simulink model "c_simulink"  (R2020a)
settings: Solver=VariableStepAuto  StartTime=0.0  StopTime=10  RelTol=1e-3
settings Model: Creator=jiw19031  LastModifiedBy=Amyang
settings OptimizationCC: BlockReduction=off  SimCompilerOptimization=on
settings ModelReferenceCC: UpdateModelReferenceTargets=Force
settings SFSimCC: SimCustomHeaderCode="#include \"tcpclient.h\""  SimUserSources=c/tcpclient.c  SimUserIncludeDirs=c/  SimUserLibraries=c/libws2_32.a  SimBuildMode=sf_nonincremental_build

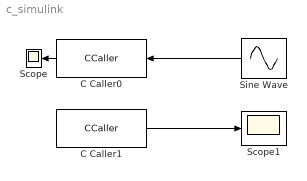
== system c_simulink ==
  C Caller0 : CCaller  FunctionName=TCPSend  PortSpecificationStruct="%)30     .    N ,   8    (     @         %    \"     (    !     0         %  0 \"0    $    _    07)G3F%M90  4&]R=$YA;64 4V-O<&4     26YD97@     5'EP90      4VEZ90      27-';&]B86P   X    P    !@    @    $          4    (     0    ,    !         !   P!O=70 #@   #     &    \"     0         !0    @    !     P    $         $  # &]U=  .    .     8    (    !          %    \"     $    &     0         0    !@   $]U='!U=   #@   #@    &    \"     8         !0    @    !     0    $         \"0    @               X    X    !@    @    $          4    (     0    8    !         !     &    9&]U8FQE   .    ,     8    (    !          %    \"     $    !     0         0  $ ,0    X    P    !@    @    ) @        4    (     0    $    !          (  0      #@   #     &    \"     0         !0    @    !     P    $         $  # &EN,  .    ,     8    (    !          %    \"     $    #     0         0  , :6XP  X    X    !@    @    $          4    (     0    4    !         !     %    26YP=70    .    .     8    (    !@         %    \"     $    !     0         )    \"               #@   #@    &    \"     0         !0    @    !    !@    $         $     8   !D;W5B;&4   X    P    !@    @    $          4    (     0    $    !         !   0 Q    #@   #     &    \"     D\"        !0    @    !     0    $          @ !"
  C Caller1 : CCaller  FunctionName=TCPRecv  PortSpecificationStruct="%)30     .    & (   8    (     @         %    \"     $    !     0         %  0 \"0    $    _    07)G3F%M90  4&]R=$YA;64 4V-O<&4     26YD97@     5'EP90      4VEZ90      27-';&]B86P   X    P    !@    @    $          4    (     0    ,    !         !   P!O=70 #@   #     &    \"     0         !0    @    !     P    $         $  # &]U=  .    .     8    (    !          %    \"     $    &     0         0    !@   $]U='!U=   #@   #@    &    \"     8         !0    @    !     0    $         \"0    @               X    X    !@    @    $          4    (     0    8    !         !     &    9&]U8FQE   .    ,     8    (    !          %    \"     $    !     0         0  $ ,0    X    P    !@    @    ) @        4    (     0    $    !          (  0"
  Scope : Scope
  Scope1 : Scope
  Sine Wave : Sin  SineType=Sample based  SampleTime=1
  wires:
  C Caller0/1 -> Scope/1
  Sine Wave/1 -> C Caller0/1
  C Caller1/1 -> Scope1/1
